simulink model "drones_simulation"  (R2025b)
settings: Solver=ode4  StartTime=0.0  StopTime=t_sim  FixedStep=Ts  RelTol=1e-3
values from neighbouring files (symbols this model uses):
  adj_row_1 = Adj_mat(1,:)    [Parameters_scenarios.m]
  adj_row_2 = Adj_mat(2,:)    [Parameters_scenarios.m]
  adj_row_3 = Adj_mat(3,:)    [Parameters_scenarios.m]
  adj_row_4 = Adj_mat(4,:)    [Parameters_scenarios.m]
  gamma1 = 8.0    (= 8)    [Parameters_scenarios.m]
  gamma2 = 8.0    (= 8)    [Parameters_scenarios.m]
  goal_tolerance = 0.05    [Parameters_scenarios.m]
  Ib = diag([Jxx, Jyy, Jzz])    [Parameters_scenarios.m]
  Kd = 2.5    [Parameters_scenarios.m]
  Kp = 1.2    [Parameters_scenarios.m]
  mass = 0.032    [Parameters_scenarios.m]
  max_acc = 2.5    [Parameters_scenarios.m]
  max_vel = 1.2 * (dist_total / desired_flight_time)    [Parameters_scenarios.m]
  Rc = 2.0    (= 2)    [Parameters_scenarios.m]
  Rs = Rs_safe    (= 0.15)    [Parameters_scenarios.m]
  Rs_obs = radius_robots + radii_obstacles + margin    (= 0.95)    [Parameters_scenarios.m]
  v0_1 = v0(1,:)'    [Parameters_scenarios.m]
  v0_2 = v0(2,:)'    [Parameters_scenarios.m]
  v0_3 = v0(3,:)'    [Parameters_scenarios.m]
  v0_4 = v0(4,:)'    [Parameters_scenarios.m]
  x0_1 = x0(1,:)'    [Parameters_scenarios.m]
  x0_2 = x0(2,:)'    [Parameters_scenarios.m]
  x0_3 = x0(3,:)'    [Parameters_scenarios.m]
  x0_4 = x0(4,:)'    [Parameters_scenarios.m]
  x_objects = [0.0 ... (first row only)    [Parameters_scenarios.m]
  xg_1 = xg(1,:)'    [Parameters_scenarios.m]
  xg_2 = xg(2,:)'    [Parameters_scenarios.m]
  xg_3 = xg(3,:)'    [Parameters_scenarios.m]
  xg_4 = xg(4,:)'    [Parameters_scenarios.m]
  xg_vec = reshape(xg', [], 1)    [Parameters_scenarios.m]
libraries: robotcorelib x4
(part 3 of 3)

== matlab function drones_simulation/MATLAB Function5 ==
  data: x_i input; v_i input; u_gtg output; xg_i input; Kp input; Kd input; max_acc input; max_vel input
function u_gtg = controller_generic(x_i, v_i, xg_i, Kp, Kd, max_acc, max_vel)

    % Errore posizione
    e_p = xg_i - x_i;
    
    % Velocità Desiderata (Proporzionale all'errore)
    % Il termine Kp * e_p è idealmente la velocità che vorremmo avere
    
    v_des = (Kp / Kd) * e_p; % velocità proporzionale all'errore di posizione
    
    % Saturazione della velocità desiderata 
    v_norm = norm(v_des);
    if v_norm > max_vel
        v_des = (v_des / v_norm) * max_vel;
    end
    
    % Controllo dove si insegue la velocità
    u_unclamped = Kd * (v_des - v_i); % equivalente a un PD classico u = Kp*ep - Kd*v
    
    % 4. Saturazione accelerazione 
    norm_u = norm(u_unclamped);
    if norm_u > max_acc
        u_gtg = (u_unclamped / norm_u) * max_acc;
    else
        u_gtg = u_unclamped;
    end
end

== matlab function drones_simulation/MATLAB Function6 ==
  data: x_i input; v_i input; u_gtg output; xg_i input; Kp input; Kd input; max_acc input; max_vel input
function u_gtg = controller_generic(x_i, v_i, xg_i, Kp, Kd, max_acc, max_vel)

    % Errore posizione
    e_p = xg_i - x_i;
    
    % Velocità Desiderata (Proporzionale all'errore)
    % Il termine Kp * e_p è idealmente la velocità che vorremmo avere
    
    v_des = (Kp / Kd) * e_p; % velocità proporzionale all'errore di posizione
    
    % Saturazione della velocità desiderata 
    v_norm = norm(v_des);
    if v_norm > max_vel
        v_des = (v_des / v_norm) * max_vel;
    end
    
    % Controllo dove si insegue la velocità
    u_unclamped = Kd * (v_des - v_i); % equivalente a un PD classico u = Kp*ep - Kd*v
    
    % 4. Saturazione accelerazione 
    norm_u = norm(u_unclamped);
    if norm_u > max_acc
        u_gtg = (u_unclamped / norm_u) * max_acc;
    else
        u_gtg = u_unclamped;
    end
end
